simulink model "foucaultStart"  (R2018a)
settings: Solver=ode23t  StartTime=0.0  StopTime=3600  FixedStep=.1  RelTol=1e-5  EnableMultiTasking=on
PreLoadFcn:
  | g = 9.83;          % acceleration of gravity (m/sec^2)
  | L = 67;            % pendulum length (m)
  | initial_x = L/100; % initial x coordinate (m)
  | initial_y = 0;     % initial y coordinate (m)
  | initial_xdot = 0;  % initial x velocity (m/sec)
  | initial_ydot = 0;  % initial y velocity (m/sec)
  | Omega=2*pi/86400;  % Earth's angular velocity of rotation about its axis (rad/sec)
  | lambda=49/180*pi;  % latitude in (rad)
CloseFcn:
  | close(findobj('Tag','CloseMe'));
settings Model: Creator=The MathWorks Inc.  LastModifiedBy=austi
settings DataIOCC: SaveFormat=StructureWithTime  SaveOutput=off  SaveTime=off  SignalLoggingName=sldemo_foucault_output
settings OptimizationCC: ExpressionDepthLimit=2147483647  InitFltsAndDblsToZero=on  LifeSpan=inf
settings DebuggingCC: SaveWithParameterizedLinksMsg=none  UnderspecifiedInitializationDetection=Classic  MergeDetectMultiDrivingBlocksExec=none  SignalResolutionControl=TryResolveAllWithWarning  ParameterPrecisionLossMsg=none  FcnCallInpInsideContextMsg=warning  AllowSymbolicDim=off  StateNameClashWarn=warning  SFUnexpectedBacktrackingDiag=warning  SFNoUnconditionalDefaultTransitionDiag=warning  SFExecutionAtInitializationDiag=none
settings HardwareCC: ProdBitPerPointer=32  ProdBitPerSizeT=32  ProdBitPerPtrDiffT=32  ProdLargestAtomicFloat=None  ProdIntDivRoundTo=Undefined  ProdEndianess=Unspecified  ProdWordSize=32  ProdHWDeviceType=32-bit Generic
settings ModelReferenceCC: PropagateSignalLabelsOutOfModel=off
settings CodeAppCC: StateflowObjectComments=on
settings GRTTargetCC: TargetFcnLib=ansi_tfl_tmw.mat  TargetLangStandard=C89/C90 (ANSI)  GeneratePreprocessorConditionals=Disable all  CombineOutputUpdateFcns=off  GRTInterface=on
settings ConfigComp: CovMetricSettings=dw  CovHtmlReporting=on  CovSaveCumulativeToWorkspaceVar=on  CovSaveSingleToWorkspaceVar=on  CovExternalEMLEnable=off  CovSFcnEnable=off

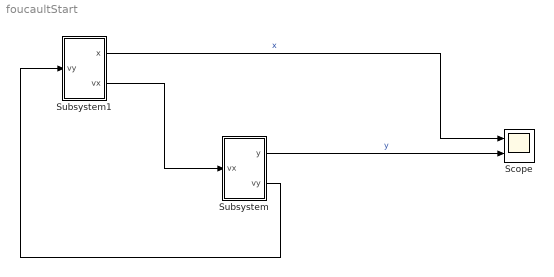
== system foucaultStart ==
  Scope : Scope  NumInputPorts=2
  Subsystem : Subsystem
  Subsystem1 : Subsystem
  wires:
  Subsystem/2(vy) -> Subsystem1/1(vy)
  Subsystem/1(y) -> Scope/2  "y"
  Subsystem1/1(x) -> Scope/1  "x"
  Subsystem1/2(vx) -> Subsystem/1(vx)

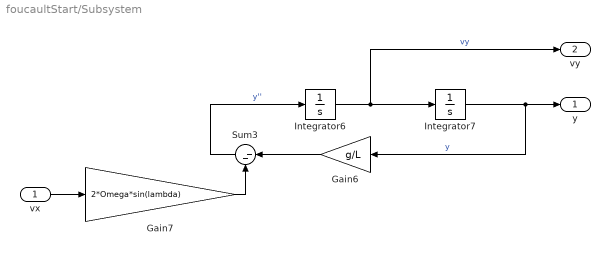
== system foucaultStart/Subsystem ==
  vx : Inport
  Gain6 : Gain  Gain=g/L
  Gain7 : Gain  Gain=2*Omega*sin(lambda)
  Integrator6 : Integrator  InitialCondition=initial_ydot
  Integrator7 : Integrator  InitialCondition=initial_y
  Sum3 : Sum  Inputs=|--
  y : Outport
  vy : Outport  Port=2
  wires:
  Gain6/1 -> Sum3/1
  vx/1 -> Gain7/1
  Integrator6/1 -> vy/1, Integrator7/1  "vy"
  Gain7/1 -> Sum3/2
  Integrator7/1 -> y/1, Gain6/1  "y"
  Sum3/1 -> Integrator6/1  "y''"

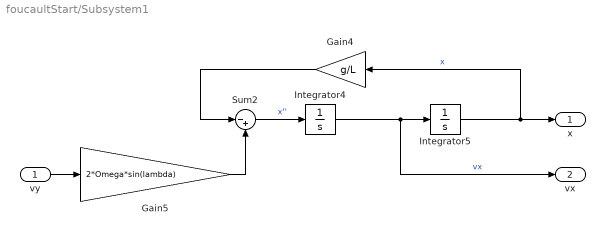
== system foucaultStart/Subsystem1 ==
  vy : Inport
  Gain4 : Gain  Gain=g/L
  Gain5 : Gain  Gain=2*Omega*sin(lambda)
  Integrator4 : Integrator  InitialCondition=initial_xdot
  Integrator5 : Integrator  InitialCondition=initial_x
  Sum2 : Sum  Inputs=|-+
  x : Outport
  vx : Outport  Port=2
  wires:
  Integrator4/1 -> vx/1, Integrator5/1  "vx"
  Sum2/1 -> Integrator4/1  "x''"
  vy/1 -> Gain5/1
  Gain5/1 -> Sum2/2
  Integrator5/1 -> x/1, Gain4/1  "x"
  Gain4/1 -> Sum2/1
